simulink model "model4"  (R2022a)
settings: Solver=VariableStepAuto  StartTime=0.0  StopTime=120  RelTol=1e-3
settings Model: Creator=tano-  LastModifiedBy=tano-

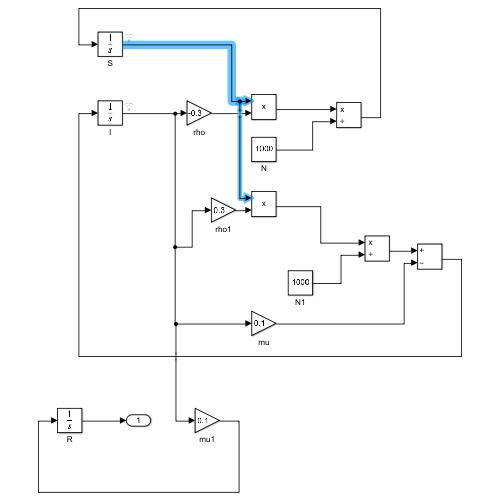
[thumbnail: Simulink's stored preview of the top-level diagram]
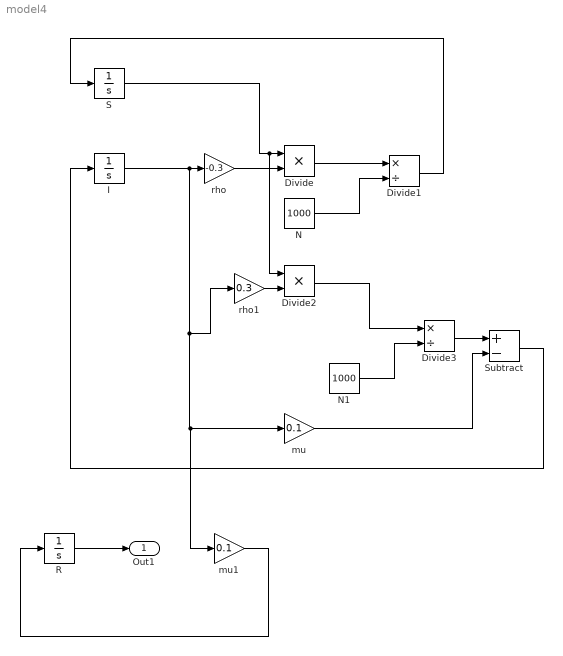
== system model4 ==
  Divide : Product  Inputs=**
  Divide1 : Product  Inputs=*/
  Divide2 : Product  Inputs=**
  Divide3 : Product  Inputs=*/
  I : Integrator  InitialCondition=2
  N : Constant  Value=1000
  N1 : Constant  Value=1000
  R : Integrator
  S : Integrator  InitialCondition=950
  Subtract : Sum  Inputs=+-
  mu : Gain  Gain=0.1
  mu1 : Gain  Gain=0.1
  rho : Gain  Gain=-0.3
  rho1 : Gain  Gain=0.3
  Out1 : Outport
  wires:
  I/1 -> rho1/1, mu/1, mu1/1, rho/1
  rho/1 -> Divide/2
  S/1 -> Divide2/1, Divide/1
  Divide/1 -> Divide1/1
  N/1 -> Divide1/2
  Divide2/1 -> Divide3/1
  N1/1 -> Divide3/2
  rho1/1 -> Divide2/2
  Divide3/1 -> Subtract/1
  mu/1 -> Subtract/2
  Divide1/1 -> S/1
  Subtract/1 -> I/1
  mu1/1 -> R/1
  R/1 -> Out1/1
